simulink model "observer_model_additional"  (R2024a)
settings: Solver=FixedStepAuto  StartTime=0.0  StopTime=1  FixedStep=0.00001  RelTol=1e-3
values from neighbouring files (symbols this model uses):
  A = [5 -5 -9 3; -5 5 -3 9; -9 -3 5 5; 3 9 5 5]    [ex.m]    (also in observer.m = [20 5 -16 9; 6 1 -4 1; 32 9 -25 14; 8 4 -6 4]; observer_down.m; reg.m = [2 3; -3 2])
  C = [1 -1 1 1; 1 3 -1 3]    [ex.m]    (also in observer.m = [-1 0 1 -1]; observer_down.m = [0 0 0 1; 0 1 0 0])
  L2 = inv(Q2)*Y2    [observer.m]
settings Model: Creator=ventus  LastModifiedBy=ventus

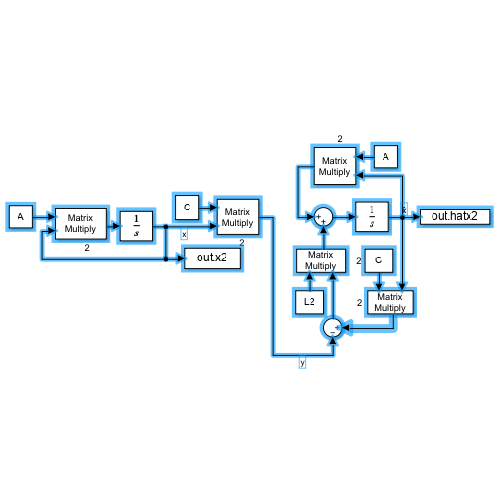
[thumbnail: Simulink's stored preview of the top-level diagram]
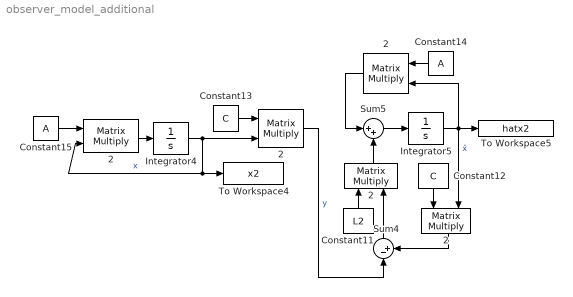
== system observer_model_additional ==
  "     2" : Product  Multiplication=Matrix(*)
  "    2" : Product  Multiplication=Matrix(*)
  "   2" : Product  Multiplication=Matrix(*)
  "  2" : Product  Multiplication=Matrix(*)
  " 2" : Product  Multiplication=Matrix(*)
  Constant11 : Constant  Value=L2  VectorParams1D=off
  Constant12 : Constant  Value=C  VectorParams1D=off
  Constant13 : Constant  Value=C  VectorParams1D=off
  Constant14 : Constant  Value=A  VectorParams1D=off
  Constant15 : Constant  Value=A  VectorParams1D=off
  Integrator4 : Integrator  InitialCondition=[1; 1; 1; 1]
  Integrator5 : Integrator  InitialCondition=[2; 0; 0; -1]
  Sum4 : Sum  Inputs=|-+
  Sum5 : Sum  Inputs=|++
  To Workspace4 : ToWorkspace  VariableName=x2  SaveFormat=Timeseries  SampleTime=-1
  To Workspace5 : ToWorkspace  VariableName=hatx2  SaveFormat=Timeseries  SampleTime=-1
  wires:
  Constant15/1 -> "     2"/1
  "    2"/1 -> Sum5/1
  "  2"/1 -> Sum5/2
  Sum4/1 -> "  2"/2
  Integrator4/1 -> "   2"/2, To Workspace4/1, "     2"/2  "x"
  Constant13/1 -> "   2"/1
  Constant11/1 -> "  2"/1
  "     2"/1 -> Integrator4/1
  Constant12/1 -> " 2"/1
  Sum5/1 -> Integrator5/1
  Integrator5/1 -> To Workspace5/1, "    2"/2, " 2"/2  "x̂"
  "   2"/1 -> Sum4/1  "y"
  Constant14/1 -> "    2"/1
  " 2"/1 -> Sum4/2
